simulink model "project"  (R2016a)
settings: Solver=VariableStepAuto  StartTime=0.0  StopTime=100  RelTol=1e-3
values from neighbouring files (symbols this model uses):
  beta = -1    [main.m]
  d = 1    [main.m]
  DT = 40    [main.m]
  Hr = [1,1]    [main.m]
  Hs = [1,-1]    [main.m]
  lambda = 0.01    [main.m]
  nA = length(A1)-1    [LPV_Torsional.m]    (also in main.m = length(G1.f)-1)
  nB = length(B1)-1    [LPV_Torsional.m]    (also in main.m = length(G1.b)-1-d)
  nr = nA + nHs + nHr -1    [main.m]
  ns = nB + nHs + nHr +d -1    [main.m]
  nt = 0    [main.m]
  Ts = 0.04    [LPV_Torsional.m]    (also in main.m = G1.Ts)
undefined symbols (not defined in the file or in its folder): G1, G2, G3, P, R1, R2, R3, S1, S2, S3
libraries: simulink x1
settings Model: Creator=grall  LastModifiedBy=grall

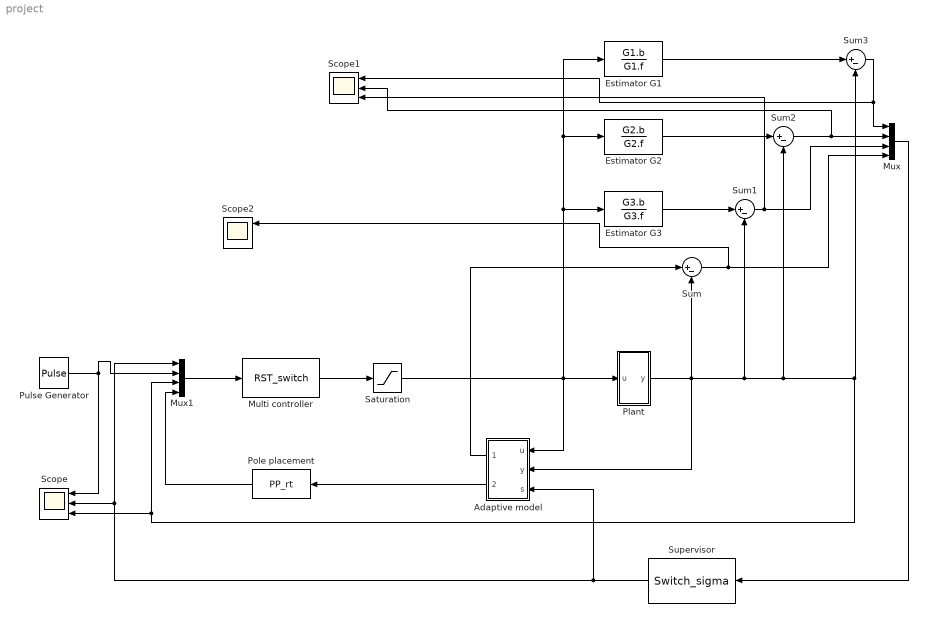
== system project ==
  Adaptive model : Subsystem
  Estimator G1 : DiscreteTransferFcn  Numerator=G1.b  Denominator=G1.f
  Estimator G2 : DiscreteTransferFcn  Numerator=G2.b  Denominator=G2.f
  Estimator G3 : DiscreteTransferFcn  Numerator=G3.b  Denominator=G3.f
  Multi controller : S-Function  FunctionName=RST_switch  Parameters=R1,S1,R2,S2,R3,S3,Ts,nr,ns,nt  SFunctionDeploymentMode=off  EnableBusSupport=off
  Mux : Mux
  Mux1 : Mux
  "Plant " : Subsystem
  Pole placement : S-Function  FunctionName=PP_rt  Parameters=nA,nB,d,P,Hs,Hr,Ts  SFunctionDeploymentMode=off  EnableBusSupport=off
  Pulse Generator : DiscretePulseGenerator  PulseType=Time based  Period=25  PulseWidth=50
  Saturation : Saturate  UpperLimit=2  LowerLimit=-2
  Scope : Scope  NumInputPorts=3
  Scope1 : Scope  NumInputPorts=3
  Scope2 : Scope  NumInputPorts=3
  Sum{,1..3} (4 alike) : Sum  Inputs=|+-
  Supervisor : S-Function  FunctionName=Switch_sigma  Parameters=beta,lambda,DT  SFunctionDeploymentMode=off  EnableBusSupport=off
  wires:
  Estimator G3/1 -> Sum1/1
  Estimator G2/1 -> Sum2/1
  Estimator G1/1 -> Sum3/1
  Sum2/1 -> Scope1/2, Mux/2
  Sum3/1 -> Scope1/1, Mux/1
  Sum1/1 -> Mux/3, Scope1/3
  Sum/1 -> Scope2/1, Mux/4
  Mux/1 -> Supervisor/1
  "Plant "/1("y ") -> Adaptive model/2(y), Sum/2, Sum2/2, Mux1/3, Scope/3, Sum3/2, Sum1/2
  Saturation/1 -> Adaptive model/1(u), Estimator G2/1, Estimator G1/1, Estimator G3/1, "Plant "/1(u)
  Adaptive model/1(yhat) -> Sum/1
  Multi controller/1 -> Saturation/1
  Adaptive model/2(theta) -> Pole placement/1
  Supervisor/1 -> Scope/2, Mux1/1, Adaptive model/3(s)
  Mux1/1 -> Multi controller/1
  Pole placement/1 -> Mux1/4
  Pulse Generator/1 -> Scope/1, Mux1/2

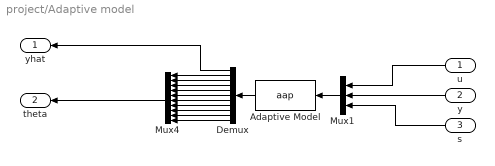
== system project/Adaptive model ==
  u : Inport
  y : Inport  Port=2
  s : Inport  Port=3
  "Adaptive Model " : S-Function  FunctionName=aap  Parameters=nA,nB,d  SFunctionDeploymentMode=off  EnableBusSupport=off
  Demux : Demux  Outputs=11
  Mux1 : Mux  Inputs=3
  Mux4 : Mux  Inputs=10
  yhat : Outport
  theta : Outport  Port=2
  wires:
  s/1 -> Mux1/3
  y/1 -> Mux1/2
  u/1 -> Mux1/1
  Demux/11 -> Mux4/10
  Demux/10 -> Mux4/9
  Demux/9 -> Mux4/8
  Demux/8 -> Mux4/7
  Demux/7 -> Mux4/6
  Demux/6 -> Mux4/5
  Demux/5 -> Mux4/4
  Demux/4 -> Mux4/3
  Demux/3 -> Mux4/2
  Demux/2 -> Mux4/1
  Mux4/1 -> theta/1
  Demux/1 -> yhat/1
  "Adaptive Model "/1 -> Demux/1
  Mux1/1 -> "Adaptive Model "/1

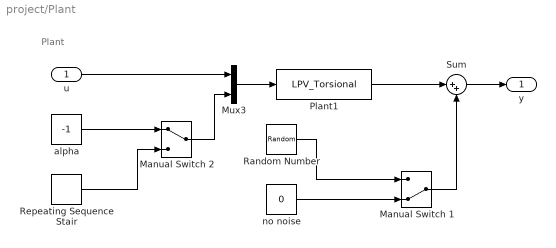
== system project/Plant  ==
  note: Plant
  u : Inport
  Manual Switch 1 : ManualSwitch  CurrentSetting=0
  Manual Switch 2 : ManualSwitch
  Mux3 : Mux  Inputs=2
  Plant1 : S-Function  FunctionName=LPV_Torsional  SFunctionDeploymentMode=off  EnableBusSupport=off
  Random Number : RandomNumber  Variance=0.00001  SampleTime=Ts
  Repeating Sequence Stair : simulink/Sources/Repeating Sequence Stair  OutValues=[-1 1 0.5 -0.5 1 0].'  tsamp=25  OutMin=[]  OutMax=[]  OutDataTypeStr=double  OutputDataTypeScalingMode=double  OutDataType=fixdt(0,8)  ConRadixGroup=Best Precision: Vector-wise  OutScaling=2^-12
  Sum : Sum  Inputs=|++
  alpha : Constant  Value=-1
  "no noise " : Constant  Value=0
  "y " : Outport
  wires:
  Sum/1 -> "y "/1
  Mux3/1 -> Plant1/1
  Plant1/1 -> Sum/1
  u/1 -> Mux3/1
  Manual Switch 2/1 -> Mux3/2
  "no noise "/1 -> Manual Switch 1/2
  Manual Switch 1/1 -> Sum/2
  Random Number/1 -> Manual Switch 1/1
  Repeating Sequence Stair/1 -> Manual Switch 2/2
  alpha/1 -> Manual Switch 2/1
